simulink model "Australian14gen_original"  (R2017a)
settings: Solver=ode23tb  StartTime=0.0  StopTime=70  MaxStep=1/60  RelTol=1e-3  AbsTol=1e-1  EnableMultiTasking=on
PreLoadFcn:
  | dataaustralian14gen
values from neighbouring files (symbols this model uses):
  bus_v = [ 101	15 ... (first row only)    [dataaustralian14gen.m]
  comp = [ 1	211	0	0 ... (first row only)    [dataaustralian14gen.m]
  Exc = [ 101	0	 200	0.1	    13.25  2.5	 0	0       0       0       0       0 ... (first row only)    [dataaustralian14gen.m]
  FH = 13    [dataaustralian14gen.m]
  FI = 1    [dataaustralian14gen.m]
  FL = .1    (= 0.1)    [dataaustralian14gen.m]
  G_data = [ 101	333.3	15	3.6	0.14	1.1	0.65	0.25	8.5     0.25	0.05	0       0       0.25	0.2 	0 ... (first row only)    [dataaustralian14gen.m]
  KH = 120    [dataaustralian14gen.m]
  KI = 10    [dataaustralian14gen.m]
  KL = 10    [dataaustralian14gen.m]
  line = [ 102	217	0.0084	0.0667	0.817	330	1 ... (first row only)    [dataaustralian14gen.m]
  p = p_case4    [dataaustralian14gen.m]
  PSSMODEL = 1    [dataaustralian14gen.m]
  trans = [ 1	101	102	15	330	333.3	12	12 ... (first row only)    [dataaustralian14gen.m]
undefined symbols (not defined in the file or in its folder): D1, Delta
libraries: powerlib x297, sps_avr x14, factslib x5, powerlib_extras x4
(part 2 of 3)

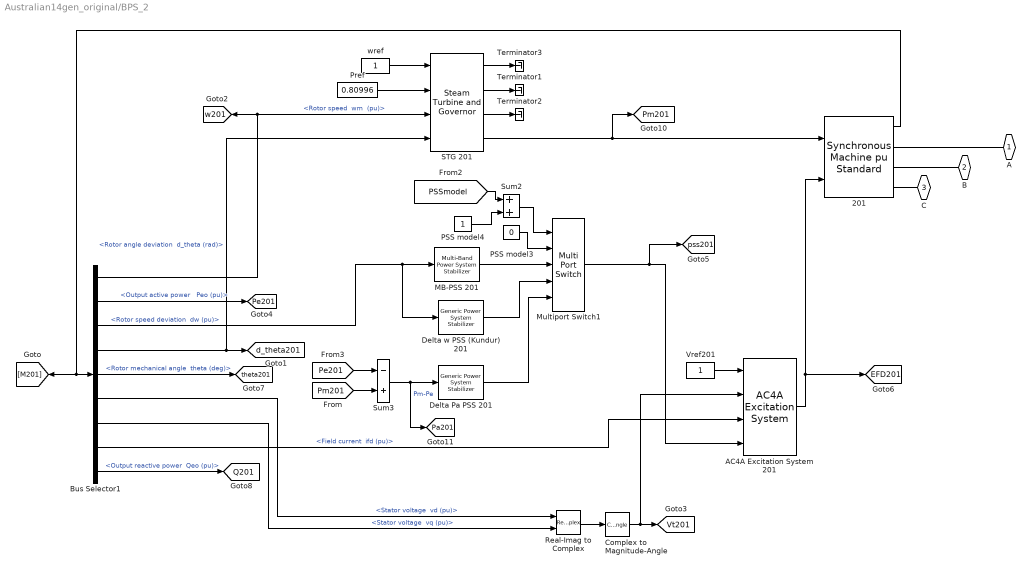
== system Australian14gen_original/BPS_2 ==
  201 : powerlib/Machines/Synchronous Machine pu Standard  PresetModel=No  MechanicalLoad=Mechanical power Pm  ShowDetailedParameters=on  RotorType=Round  Units=per unit standard parameters  MeasurementBus=off  NominalParameters="[G_data(2,2)*1e6  G_data(2,3)*1e3  50]"  Reactances1=[G_data(2,6),G_data(2,8),G_data(2,10),G_data(2,7),G_data(2,12),G_data(2,14),G_data(2,5)]  Reactances2=[G_data(2,6),G_data(2,8),G_data(2,10),G_data(2,7),G_data(2,14),G_data(2,5)]  dAxisTimeConstants=Open-circuit  qAxisTimeConstants=Open-circuit  TimeConstants1="[G_data(2,9)  G_data(2,11)  G_data(2,15)]"  TimeConstants2="[G_data(2,9), G_data(2,11), G_data(2,13),  G_data(2,15)]"  TimeConstants3="[  5.9  0.033  0.023  ]"  TimeConstants4=[ 8.0, 0.03, 0.3371, 0.0295 ]  TimeConstants5=[ 1.01, 0.053, 0.1 ]  TimeConstants6=[ 1.3201, 0.023, 1.0, 0.07 ]  TimeConstants7="[  1.01  0.053  0.051266  ]"  TimeConstants8=[ 1.3201, 0.0231, 0.3371, 0.0295 ]  StatorResistance=0  Mechanical="[ G_data(2,4) 0  4 ]"  PolePairs=4  InitialConditions=[0 -27.3285 0.811724 0.811724 0.811724 9.04729 -110.953 129.047 1.71513]  SetSaturation=off  Saturation=[0.6404,0.7127,0.8441,0.9214,0.9956,1.082,1.19,1.316,1.457;0.7,0.7698,0.8872,0.9466,0.9969,1.046,1.1,1.151,1.201]  LoadFlowParameters=[1 2160000000 20000 0 0]  TsPowergui=0  TsBlock=-1  IterativeModel=Forward Euler  IterativeDiscreteModel=Trapezoidal non iterative  BusType=PV  Pref=p(2,3)*1e6  Qref=0  Qmin=-inf  Qmax=inf  PLF=0  QLF=0
      settings: SourceProductName=Simscape Power Systems
  AC4A Excitation System 201 : sps_avr/AC4A Excitation System  Tr=Exc(2,2)  KaTa="[Exc(2,3)   Exc(2,4)]"  VIminmax=[-10 10]  VRminmax=[-4.53 5.64]  TbTc="[Exc(2,5)  Exc(2,6)]"  Kc=0  v0=[1 1.7151]  TsBlock=0
      settings: SourceProductName=Simscape Power Systems  SourceProductBaseCode=PS
  Bus Selector1 : BusSelector  OutputSignals="Mechanical.Rotor speed  wm  (pu),Output active power   Peo (pu),Mechanical.Rotor speed deviation  dw (pu),Mechanical.Rotor angle deviation  d_theta (rad),Mechanical.Rotor mechanical angle  theta (deg),dq0 components.Stator voltage  vd (pu),dq0 components.Stator voltage  vq (pu),dq0 components.Field current  ifd (pu),Output reactive power  Qeo (pu)"
  Complex to Magnitude-Angle : ComplexToMagnitudeAngle  Output=Magnitude
  Delta Pa PSS 201 : powerlib/Machines/Generic Power System Stabilizer  Tsensor=15e-3  K=2.5*1.25  Twashout=1  Tleadlag1=[60e-3 1]  Tleadlag2=[0 0]  VSlimits=[-0.15 0.15]  Vinit=0  Plot_On=off  MagdB_On=on  FreqRange=logspace(-2,2,500)
      settings: SourceProductName=Simscape Power Systems  SourceProductBaseCode=PS
  Delta w PSS (Kundur) 201 : powerlib/Machines/Generic Power System Stabilizer  Tsensor=15e-3  K=30  Twashout=10  Tleadlag1=[50e-3 20e-3]  Tleadlag2=[3 5.4]  VSlimits=[-0.15 0.15]  Vinit=0  Plot_On=off  MagdB_On=on  FreqRange=logspace(-2,2,500)
      settings: SourceProductName=Simscape Power Systems  SourceProductBaseCode=PS
  MB-PSS 201 : powerlib/Machines/Multi-Band Power System Stabilizer  OperationMode=Simplified settings  Kg=G  GL="[FL  KL]"  GI="[FI  KI]"  GH="[FH  KH]"  GLd=[66 66 9.4]  TcLF=[1.667 2 0 0 0 0 2 2.4 0 0 0 0 1 1]  GId=[66 66 47.6]  TcIF=[1 1 0.25 0.3 0 0 1 1 0.3 0.36 0 0 0 0]  GHd=[66 66 233]  TcHF="[0.01 0.012 0 0 0 0  0.012 0.0144 0 0 0 0 1 1]"  LIM=[.075 .15 .15 .15]  Plot_On=off  MagdB_On=off  FreqRange=logspace(-2,2,500)
      settings: SourceProductName=Simscape Power Systems  SourceProductBaseCode=PS
  Multiport Switch1 : MultiPortSwitch  Inputs=4  InputSameDT=on
  PSS model3 : Constant  Value=0
  PSS model4 : Constant
  Pref : Constant  Value=0.80996
  Real-Imag to Complex : RealImagToComplex
  STG 201 : powerlib/Machines/Steam Turbine and Governor  gentype=Tandem-compound (single mass)  reg1="[ 1  0.05    0 ]"  reg2="[ 0.001  0.15 ]"  reg3="[ -0.1  0.1  0  4.496 ]"  N=3000  turb1="[ 0  10   3.3   0.5   ]"  turb2="[   0   0.36    0.36   0.28   ]"  HA="[ 0.046  1.430  1.465   0.192 ]"  KA="[ 90.44  53.88  64.59   62.94  ]"  DA="[ 0.0115  0.3575  0.3663   0.0137  ]"  ini1=0.80996  ini2=[0.779316,-31.4247]
      settings: SourceProductName=Simscape Power Systems  SourceProductBaseCode=PS
  Sum2 : Sum  SaturateOnIntegerOverflow=on  InputSameDT=on  OutDataTypeStr=Inherit: Same as first input
  Sum3 : Sum  Inputs=-+  SaturateOnIntegerOverflow=on  InputSameDT=on  OutDataTypeStr=Inherit: Same as first input
  Terminator1 : Terminator
  Terminator2 : Terminator
  Terminator3 : Terminator
  Vref201 : Constant
  wref : Constant
  A : PMIOPort  Port=1  Side=Left
  B : PMIOPort  Port=2  Side=Left
  C : PMIOPort  Port=3  Side=Left
  tag scope: EFD201=global, Pa201=global, Pe201=global, Pm201=global, Q201=global, Vt201=global, d_theta201=global, pss201=global, theta201=global, w201=global
  wires:
  Bus Selector1/7 -> Real-Imag to Complex/2  "<Stator voltage  vq (pu)>"
  Bus Selector1/6 -> Real-Imag to Complex/1  "<Stator voltage  vd (pu)>"
  wref/1 -> STG 201/1
  Vref201/1 -> AC4A Excitation System 201/1
  Bus Selector1/4 -> STG 201/4, [d_theta201]  "<Rotor angle deviation  d_theta (rad)>"
  201/1 -> Bus Selector1/1, [M201]
  Bus Selector1/1 -> [w201], STG 201/3  "<Rotor speed  wm  (pu)>"
  Bus Selector1/3 -> Delta w PSS (Kundur) 201/1, MB-PSS 201/1  "<Rotor speed deviation  dw (pu)>"
  Real-Imag to Complex/1 -> Complex to Magnitude-Angle/1
  Complex to Magnitude-Angle/1 -> AC4A Excitation System 201/2, [Vt201]
  AC4A Excitation System 201/1 -> 201/2, [EFD201]
  Multiport Switch1/1 -> [pss201], AC4A Excitation System 201/4
  Bus Selector1/5 -> [theta201]  "<Rotor mechanical angle  theta (deg)>"
  Bus Selector1/2 -> [Pe201]  "<Output active power   Peo (pu)>"
  Bus Selector1/8 -> AC4A Excitation System 201/3  "<Field current  ifd (pu)>"
  Pref/1 -> STG 201/2
  STG 201/4 -> [Pm201], 201/1
  Bus Selector1/9 -> [Q201]  "<Output reactive power  Qeo (pu)>"
  PSS model4/1 -> Sum2/2
  Sum2/1 -> Multiport Switch1/1
  [PSSmodel] -> Sum2/1
  PSS model3/1 -> Multiport Switch1/2
  Sum3/1 -> [Pa201], Delta Pa PSS 201/1  "Pm-Pe"
  Delta Pa PSS 201/1 -> Multiport Switch1/5
  Delta w PSS (Kundur) 201/1 -> Multiport Switch1/4
  [Pm201] -> Sum3/2
  [Pe201] -> Sum3/1
  MB-PSS 201/1 -> Multiport Switch1/3
  STG 201/1 -> Terminator3/1
  STG 201/2 -> Terminator1/1
  STG 201/3 -> Terminator2/1
  connections:
  201/RConn1 -- A/RConn1
  201/RConn2 -- B/RConn1
  201/RConn3 -- C/RConn1

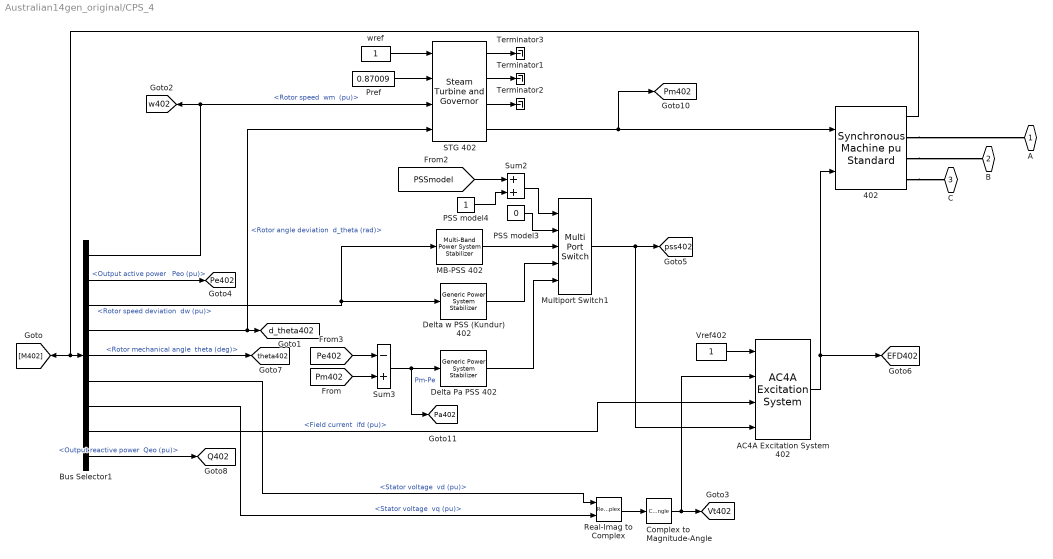
== system Australian14gen_original/CPS_4 ==
  402 : powerlib/Machines/Synchronous Machine pu Standard  PresetModel=No  MechanicalLoad=Mechanical power Pm  ShowDetailedParameters=on  RotorType=Round  Units=per unit standard parameters  MeasurementBus=off  NominalParameters="[G_data(9,2)*1e6  G_data(9,3)*1e3  50]"  Reactances1=[G_data(9,6),G_data(9,8),G_data(9,10),G_data(9,7),G_data(9,12),G_data(9,14),G_data(9,5)]  Reactances2=[G_data(9,6),G_data(9,8),G_data(9,10),G_data(9,7),G_data(9,14),G_data(9,5)]  dAxisTimeConstants=Open-circuit  qAxisTimeConstants=Open-circuit  TimeConstants1="[G_data(9,9)  G_data(9,11)  G_data(9,15)]"  TimeConstants2="[G_data(9,9)  G_data(9,11)  G_data(9,13)  G_data(9,15)]"  TimeConstants3="[  5.9  0.033  0.023  ]"  TimeConstants4=[ 8.0, 0.03, 0.3371, 0.0295 ]  TimeConstants5=[ 1.01, 0.053, 0.1 ]  TimeConstants6=[ 1.3201, 0.023, 1.0, 0.07 ]  TimeConstants7="[  1.01  0.053  0.051266  ]"  TimeConstants8=[ 1.3201, 0.0231, 0.3371, 0.0295 ]  StatorResistance=0  Mechanical="[ G_data(9,4) 0  4 ]"  PolePairs=4  InitialConditions=[0 -31.211 0.87022 0.87022 0.87022 1.63211 -118.368 121.632 1.91669]  SetSaturation=off  Saturation=[0.6404,0.7127,0.8441,0.9214,0.9956,1.082,1.19,1.316,1.457;0.7,0.7698,0.8872,0.9466,0.9969,1.046,1.1,1.151,1.201]  LoadFlowParameters=[1 580000000 20000 0 0]  TsPowergui=0  TsBlock=-1  IterativeModel=Forward Euler  IterativeDiscreteModel=Trapezoidal non iterative  BusType=PV  Pref=p(9,3)*1e6  Qref=0  Qmin=-inf  Qmax=inf  PLF=0  QLF=0
      settings: SourceProductName=Simscape Power Systems
  AC4A Excitation System 402 : sps_avr/AC4A Excitation System  Tr=Exc(9,2)  KaTa="[Exc(9,3)   Exc(9,4)]"  VIminmax=[-10 10]  VRminmax=[-4.53 5.64]  TbTc="[Exc(9,5)  Exc(9,6)]"  Kc=0  v0=[1 1.9167]  TsBlock=0
      settings: SourceProductName=Simscape Power Systems  SourceProductBaseCode=PS
  Bus Selector1 : BusSelector  OutputSignals="Mechanical.Rotor speed  wm  (pu),Output active power   Peo (pu),Mechanical.Rotor speed deviation  dw (pu),Mechanical.Rotor angle deviation  d_theta (rad),Mechanical.Rotor mechanical angle  theta (deg),dq0 components.Stator voltage  vd (pu),dq0 components.Stator voltage  vq (pu),dq0 components.Field current  ifd (pu),Output reactive power  Qeo (pu)"
  Complex to Magnitude-Angle : ComplexToMagnitudeAngle  Output=Magnitude
  Delta Pa PSS 402 : powerlib/Machines/Generic Power System Stabilizer  Tsensor=15e-3  K=2.5*1.25  Twashout=1  Tleadlag1=[60e-3 1]  Tleadlag2=[0 0]  VSlimits=[-0.15 0.15]  Vinit=0  Plot_On=off  MagdB_On=on  FreqRange=logspace(-2,2,500)
      settings: SourceProductName=Simscape Power Systems  SourceProductBaseCode=PS
  Delta w PSS (Kundur) 402 : powerlib/Machines/Generic Power System Stabilizer  Tsensor=15e-3  K=30  Twashout=10  Tleadlag1=[50e-3 20e-3]  Tleadlag2=[3 5.4]  VSlimits=[-0.15 0.15]  Vinit=0  Plot_On=off  MagdB_On=on  FreqRange=logspace(-2,2,500)
      settings: SourceProductName=Simscape Power Systems  SourceProductBaseCode=PS
  MB-PSS 402 : powerlib/Machines/Multi-Band Power System Stabilizer  OperationMode=Simplified settings  Kg=G  GL="[FL  KL]"  GI="[FI  KI]"  GH="[FH  KH]"  GLd=[66 66 9.4]  TcLF=[1.667 2 0 0 0 0 2 2.4 0 0 0 0 1 1]  GId=[66 66 47.6]  TcIF=[1 1 0.25 0.3 0 0 1 1 0.3 0.36 0 0 0 0]  GHd=[66 66 233]  TcHF="[0.01 0.012 0 0 0 0  0.012 0.0144 0 0 0 0 1 1]"  LIM=[.075 .15 .15 .15]  Plot_On=off  MagdB_On=off  FreqRange=logspace(-2,2,500)
      settings: SourceProductName=Simscape Power Systems  SourceProductBaseCode=PS
  Multiport Switch1 : MultiPortSwitch  Inputs=4  InputSameDT=on
  PSS model3 : Constant  Value=0
  PSS model4 : Constant
  Pref : Constant  Value=0.87009
  Real-Imag to Complex : RealImagToComplex
  STG 402 : powerlib/Machines/Steam Turbine and Governor  gentype=Tandem-compound (single mass)  reg1="[ 1  0.05    0 ]"  reg2="[ 0.001  0.15 ]"  reg3="[ -0.1  0.1  0  4.496 ]"  N=3000  turb1="[ 0  10   3.3   0.5   ]"  turb2="[   0   0.36    0.36   0.28   ]"  HA="[ 0.046  1.430  1.465   0.192 ]"  KA="[ 90.44  53.88  64.59   62.94  ]"  DA="[ 0.0115  0.3575  0.3663   0.0137  ]"  ini1=0.87009  ini2=[0.779316,-31.4247]
      settings: SourceProductName=Simscape Power Systems  SourceProductBaseCode=PS
  Sum2 : Sum  SaturateOnIntegerOverflow=on  InputSameDT=on  OutDataTypeStr=Inherit: Same as first input
  Sum3 : Sum  Inputs=-+  SaturateOnIntegerOverflow=on  InputSameDT=on  OutDataTypeStr=Inherit: Same as first input
  Terminator1 : Terminator
  Terminator2 : Terminator
  Terminator3 : Terminator
  Vref402 : Constant
  wref : Constant
  A : PMIOPort  Port=1  Side=Left
  B : PMIOPort  Port=2  Side=Left
  C : PMIOPort  Port=3  Side=Left
  tag scope: EFD402=global, Pa402=global, Pe402=global, Pm402=global, Q402=global, Vt402=global, d_theta402=global, pss402=global, theta402=global, w402=global
  wires:
  Bus Selector1/7 -> Real-Imag to Complex/2  "<Stator voltage  vq (pu)>"
  Bus Selector1/6 -> Real-Imag to Complex/1  "<Stator voltage  vd (pu)>"
  wref/1 -> STG 402/1
  Vref402/1 -> AC4A Excitation System 402/1
  Bus Selector1/4 -> STG 402/4, [d_theta402]  "<Rotor angle deviation  d_theta (rad)>"
  402/1 -> Bus Selector1/1, [M402]
  Bus Selector1/1 -> [w402], STG 402/3  "<Rotor speed  wm  (pu)>"
  Bus Selector1/3 -> Delta w PSS (Kundur) 402/1, MB-PSS 402/1  "<Rotor speed deviation  dw (pu)>"
  Real-Imag to Complex/1 -> Complex to Magnitude-Angle/1
  Complex to Magnitude-Angle/1 -> AC4A Excitation System 402/2, [Vt402]
  AC4A Excitation System 402/1 -> 402/2, [EFD402]
  Multiport Switch1/1 -> AC4A Excitation System 402/4, [pss402]
  Bus Selector1/5 -> [theta402]  "<Rotor mechanical angle  theta (deg)>"
  Bus Selector1/2 -> [Pe402]  "<Output active power   Peo (pu)>"
  Bus Selector1/8 -> AC4A Excitation System 402/3  "<Field current  ifd (pu)>"
  Pref/1 -> STG 402/2
  STG 402/4 -> [Pm402], 402/1
  Bus Selector1/9 -> [Q402]  "<Output reactive power  Qeo (pu)>"
  PSS model4/1 -> Sum2/2
  Sum2/1 -> Multiport Switch1/1
  [PSSmodel] -> Sum2/1
  PSS model3/1 -> Multiport Switch1/2
  Sum3/1 -> [Pa402], Delta Pa PSS 402/1  "Pm-Pe"
  Delta Pa PSS 402/1 -> Multiport Switch1/5
  Delta w PSS (Kundur) 402/1 -> Multiport Switch1/4
  [Pm402] -> Sum3/2
  [Pe402] -> Sum3/1
  MB-PSS 402/1 -> Multiport Switch1/3
  STG 402/1 -> Terminator3/1
  STG 402/2 -> Terminator1/1
  STG 402/3 -> Terminator2/1
  connections:
  402/RConn1 -- A/RConn1
  402/RConn2 -- B/RConn1
  402/RConn3 -- C/RConn1

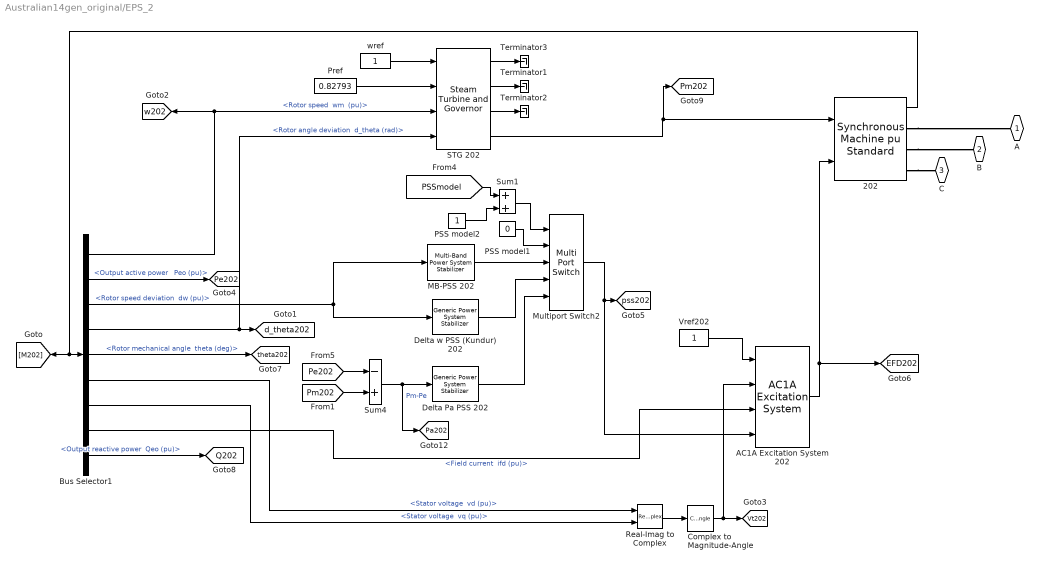
== system Australian14gen_original/EPS_2 ==
  202 : powerlib/Machines/Synchronous Machine pu Standard  PresetModel=No  MechanicalLoad=Mechanical power Pm  ShowDetailedParameters=on  RotorType=Round  Units=per unit standard parameters  MeasurementBus=off  NominalParameters="[G_data(3,2)*1e6  G_data(3,3)*1e3  50]"  Reactances1=[G_data(3,6),G_data(3,8),G_data(3,10),G_data(3,7),G_data(3,12), G_data(3,14),G_data(3,5)]  Reactances2=[G_data(3,6),G_data(3,8),G_data(3,10),G_data(3,7),G_data(3,12), G_data(3,14),G_data(3,5)]  dAxisTimeConstants=Open-circuit  qAxisTimeConstants=Open-circuit  TimeConstants1="[G_data(3,9)  G_data(3,11)  G_data(3,13) G_data(3,15)]"  TimeConstants2="[G_data(3,9)  G_data(3,11)  G_data(3,13) G_data(3,15)]"  TimeConstants3="[  5.9  0.033  0.023  ]"  TimeConstants4=[ 8.0, 0.03, 0.3371, 0.0295 ]  TimeConstants5=[ 1.01, 0.053, 0.1 ]  TimeConstants6=[ 1.3201, 0.023, 1.0, 0.07 ]  TimeConstants7="[  1.01  0.053  0.051266  ]"  TimeConstants8=[ 1.3201, 0.0231, 0.3371, 0.0295 ]  StatorResistance=0  Mechanical="[ G_data(3,4) 0  4 ]"  PolePairs=4  InitialConditions=[0 -27.8373 0.828196 0.828196 0.828196 2.41486 -117.585 122.415 2.0558]  SetSaturation=off  Saturation=[0.6404,0.7127,0.8441,0.9214,0.9956,1.082,1.19,1.316,1.457;0.7,0.7698,0.8872,0.9466,0.9969,1.046,1.1,1.151,1.201]  LoadFlowParameters=[1 1380000000 20000 0 0]  TsPowergui=0  TsBlock=-1  IterativeModel=Forward Euler  IterativeDiscreteModel=Trapezoidal non iterative  BusType=PV  Pref=p(3,3)*1e6  Qref=0  Qmin=-inf  Qmax=inf  PLF=0  QLF=0
      settings: SourceProductName=Simscape Power Systems
  AC1A Excitation System 202 : sps_avr/AC1A Excitation System  Tr=Exc(3,2)  KaTa="[Exc(3,3)   Exc(3,4)]"  VAminmax=[-14.5 14.5]  VRminmax=[-5.43 6.03]  KfTf="[Exc(3,9)  Exc(3,10)]"  TbTc="[Exc(3,5)  Exc(3,6)]"  KeTe="[Exc(3,7)  Exc(3,8)]"  Ve12=[4.18 3.14]  SeVe12=[0.10 0.03]  Kd=0.38  Kc=0.20  v0=[1 2.0558]  TsBlock=0
      settings: SourceProductName=Simscape Power Systems  SourceProductBaseCode=PS
  Bus Selector1 : BusSelector  OutputSignals="Mechanical.Rotor speed  wm  (pu),Output active power   Peo (pu),Mechanical.Rotor speed deviation  dw (pu),Mechanical.Rotor angle deviation  d_theta (rad),Mechanical.Rotor mechanical angle  theta (deg),dq0 components.Stator voltage  vd (pu),dq0 components.Stator voltage  vq (pu),dq0 components.Field current  ifd (pu),Output reactive power  Qeo (pu)"
  Complex to Magnitude-Angle : ComplexToMagnitudeAngle  Output=Magnitude
  Delta Pa PSS 202 : powerlib/Machines/Generic Power System Stabilizer  Tsensor=15e-3  K=2.5*1.25  Twashout=1  Tleadlag1=[60e-3 1]  Tleadlag2=[0 0]  VSlimits=[-0.15 0.15]  Vinit=0  Plot_On=off  MagdB_On=on  FreqRange=logspace(-2,2,500)
      settings: SourceProductName=Simscape Power Systems  SourceProductBaseCode=PS
  Delta w PSS (Kundur) 202 : powerlib/Machines/Generic Power System Stabilizer  Tsensor=15e-3  K=30  Twashout=10  Tleadlag1=[50e-3 20e-3]  Tleadlag2=[3 5.4]  VSlimits=[-0.15 0.15]  Vinit=0  Plot_On=off  MagdB_On=on  FreqRange=logspace(-2,2,500)
      settings: SourceProductName=Simscape Power Systems  SourceProductBaseCode=PS
  MB-PSS 202 : powerlib/Machines/Multi-Band Power System Stabilizer  OperationMode=Simplified settings  Kg=G  GL="[FL  KL]"  GI="[FI  KI]"  GH="[FH  KH]"  GLd=[66 66 9.4]  TcLF=[1.667 2 0 0 0 0 2 2.4 0 0 0 0 1 1]  GId=[66 66 47.6]  TcIF=[1 1 0.25 0.3 0 0 1 1 0.3 0.36 0 0 0 0]  GHd=[66 66 233]  TcHF="[0.01 0.012 0 0 0 0  0.012 0.0144 0 0 0 0 1 1]"  LIM=[.075 .15 .15 .15]  Plot_On=off  MagdB_On=off  FreqRange=logspace(-2,2,500)
      settings: SourceProductName=Simscape Power Systems  SourceProductBaseCode=PS
  Multiport Switch2 : MultiPortSwitch  Inputs=4  InputSameDT=on
  PSS model1 : Constant  Value=0
  PSS model2 : Constant
  Pref : Constant  Value=0.82793
  Real-Imag to Complex : RealImagToComplex
  STG 202 : powerlib/Machines/Steam Turbine and Governor  gentype=Tandem-compound (single mass)  reg1="[ 1  0.05    0 ]"  reg2="[ 0.001  0.15 ]"  reg3="[ -0.1  0.1  0  4.496 ]"  N=3000  turb1="[ 0  10   3.3   0.5   ]"  turb2="[   0   0.36    0.36   0.28   ]"  HA="[ 0.046  1.430  1.465   0.192 ]"  KA="[ 90.44  53.88  64.59   62.94  ]"  DA="[ 0.0115  0.3575  0.3663   0.0137  ]"  ini1=0.82793  ini2=[0.779316,-31.4247]
      settings: SourceProductName=Simscape Power Systems  SourceProductBaseCode=PS
  Sum1 : Sum  SaturateOnIntegerOverflow=on  InputSameDT=on  OutDataTypeStr=Inherit: Same as first input
  Sum4 : Sum  Inputs=-+  SaturateOnIntegerOverflow=on  InputSameDT=on  OutDataTypeStr=Inherit: Same as first input
  Terminator1 : Terminator
  Terminator2 : Terminator
  Terminator3 : Terminator
  Vref202 : Constant
  wref : Constant
  A : PMIOPort  Port=1  Side=Left
  B : PMIOPort  Port=2  Side=Left
  C : PMIOPort  Port=3  Side=Left
  tag scope: EFD202=global, Pa202=global, Pe202=global, Pm202=global, Q202=global, Vt202=global, d_theta202=global, pss202=global, theta202=global, w202=global
  wires:
  Bus Selector1/7 -> Real-Imag to Complex/2  "<Stator voltage  vq (pu)>"
  Bus Selector1/6 -> Real-Imag to Complex/1  "<Stator voltage  vd (pu)>"
  wref/1 -> STG 202/1
  Vref202/1 -> AC1A Excitation System 202/1
  Bus Selector1/4 -> STG 202/4, [d_theta202]  "<Rotor angle deviation  d_theta (rad)>"
  202/1 -> [M202], Bus Selector1/1
  Bus Selector1/1 -> STG 202/3, [w202]  "<Rotor speed  wm  (pu)>"
  Bus Selector1/3 -> MB-PSS 202/1, Delta w PSS (Kundur) 202/1  "<Rotor speed deviation  dw (pu)>"
  Real-Imag to Complex/1 -> Complex to Magnitude-Angle/1
  Complex to Magnitude-Angle/1 -> AC1A Excitation System 202/2, [Vt202]
  AC1A Excitation System 202/1 -> 202/2, [EFD202]
  Multiport Switch2/1 -> AC1A Excitation System 202/4, [pss202]
  Bus Selector1/5 -> [theta202]  "<Rotor mechanical angle  theta (deg)>"
  Bus Selector1/2 -> [Pe202]  "<Output active power   Peo (pu)>"
  Bus Selector1/8 -> AC1A Excitation System 202/3  "<Field current  ifd (pu)>"
  Pref/1 -> STG 202/2
  STG 202/4 -> [Pm202], 202/1
  Bus Selector1/9 -> [Q202]  "<Output reactive power  Qeo (pu)>"
  PSS model2/1 -> Sum1/2
  Sum1/1 -> Multiport Switch2/1
  [PSSmodel] -> Sum1/1
  PSS model1/1 -> Multiport Switch2/2
  Sum4/1 -> [Pa202], Delta Pa PSS 202/1  "Pm-Pe"
  Delta Pa PSS 202/1 -> Multiport Switch2/5
  Delta w PSS (Kundur) 202/1 -> Multiport Switch2/4
  [Pm202] -> Sum4/2
  [Pe202] -> Sum4/1
  MB-PSS 202/1 -> Multiport Switch2/3
  STG 202/1 -> Terminator3/1
  STG 202/2 -> Terminator1/1
  STG 202/3 -> Terminator2/1
  connections:
  202/RConn1 -- A/RConn1
  202/RConn2 -- B/RConn1
  202/RConn3 -- C/RConn1

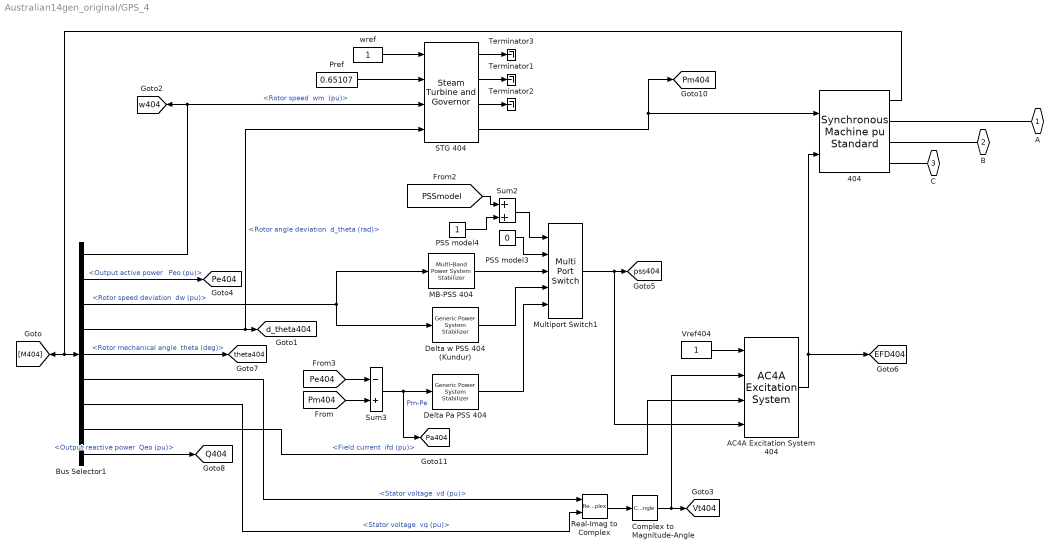
== system Australian14gen_original/GPS_4 ==
  404 : powerlib/Machines/Synchronous Machine pu Standard  PresetModel=No  MechanicalLoad=Mechanical power Pm  ShowDetailedParameters=on  RotorType=Round  Units=per unit standard parameters  MeasurementBus=off  NominalParameters="[G_data(11,2)*1e6  G_data(11,3)*1e3  50]"  Reactances1="[G_data(11,6),G_data(11,8),G_data(11,10),G_data(11,7),  G_data(11,12),G_data(11,14),G_data(11,5)]"  Reactances2="[G_data(11,6),G_data(11,8),G_data(11,10),G_data(11,7),  G_data(11,12),G_data(11,14),G_data(11,5)]"  dAxisTimeConstants=Open-circuit  qAxisTimeConstants=Open-circuit  TimeConstants1="[G_data(11,9)  G_data(11,11)   G_data(11,13) G_data(11,15)]"  TimeConstants2="[G_data(11,9)  G_data(11,11)   G_data(11,13)  G_data(11,15)]"  TimeConstants3="[  5.9  0.033  0.023  ]"  TimeConstants4=[ 8.0, 0.03, 0.3371, 0.0295 ]  TimeConstants5=[ 1.01, 0.053, 0.1 ]  TimeConstants6=[ 1.3201, 0.023, 1.0, 0.07 ]  TimeConstants7="[  1.01  0.053  0.051266  ]"  TimeConstants8=[ 1.3201, 0.0231, 0.3371, 0.0295 ]  StatorResistance=0  Mechanical="[ G_data(11,4) 0  4 ]"  PolePairs=4  InitialConditions=[0 -53.1224 0.651374 0.651374 0.651374 -4.51974 -124.52 115.48 1.67704]  SetSaturation=off  Saturation=[0.6404,0.7127,0.8441,0.9214,0.9956,1.082,1.19,1.316,1.457;0.7,0.7698,0.8872,0.9466,0.9969,1.046,1.1,1.151,1.201]  LoadFlowParameters=[1 651000000 20000 0 0]  TsPowergui=0  TsBlock=-1  IterativeModel=Forward Euler  IterativeDiscreteModel=Trapezoidal non iterative  BusType=PV  Pref=p(11,3)*1e6  Qref=0  Qmin=-inf  Qmax=inf  PLF=0  QLF=0
      settings: SourceProductName=Simscape Power Systems
  AC4A Excitation System 404 : sps_avr/AC4A Excitation System  Tr=Exc(11,2)  KaTa="[Exc(11,3)   Exc(11,4)]"  VIminmax=[-10 10]  VRminmax=[-4.53 5.64]  TbTc="[Exc(11,5)  Exc(11,6)]"  Kc=0  v0=[1 1.677]  TsBlock=0
      settings: SourceProductName=Simscape Power Systems  SourceProductBaseCode=PS
  Bus Selector1 : BusSelector  OutputSignals="Mechanical.Rotor speed  wm  (pu),Output active power   Peo (pu),Mechanical.Rotor speed deviation  dw (pu),Mechanical.Rotor angle deviation  d_theta (rad),Mechanical.Rotor mechanical angle  theta (deg),dq0 components.Stator voltage  vd (pu),dq0 components.Stator voltage  vq (pu),dq0 components.Field current  ifd (pu),Output reactive power  Qeo (pu)"
  Complex to Magnitude-Angle : ComplexToMagnitudeAngle  Output=Magnitude
  "Delta Pa PSS 404 " : powerlib/Machines/Generic Power System Stabilizer  Tsensor=15e-3  K=2.5*1.25  Twashout=1  Tleadlag1=[60e-3 1]  Tleadlag2=[0 0]  VSlimits=[-0.15 0.15]  Vinit=0  Plot_On=off  MagdB_On=on  FreqRange=logspace(-2,2,500)
      settings: SourceProductName=Simscape Power Systems  SourceProductBaseCode=PS
  "Delta w PSS 404 (Kundur) " : powerlib/Machines/Generic Power System Stabilizer  Tsensor=15e-3  K=30  Twashout=10  Tleadlag1=[50e-3 20e-3]  Tleadlag2=[3 5.4]  VSlimits=[-0.15 0.15]  Vinit=0  Plot_On=off  MagdB_On=on  FreqRange=logspace(-2,2,500)
      settings: SourceProductName=Simscape Power Systems  SourceProductBaseCode=PS
  "MB-PSS 404 " : powerlib/Machines/Multi-Band Power System Stabilizer  OperationMode=Simplified settings  Kg=G  GL="[FL  KL]"  GI="[FI  KI]"  GH="[FH  KH]"  GLd=[66 66 9.4]  TcLF=[1.667 2 0 0 0 0 2 2.4 0 0 0 0 1 1]  GId=[66 66 47.6]  TcIF=[1 1 0.25 0.3 0 0 1 1 0.3 0.36 0 0 0 0]  GHd=[66 66 233]  TcHF="[0.01 0.012 0 0 0 0  0.012 0.0144 0 0 0 0 1 1]"  LIM=[.075 .15 .15 .15]  Plot_On=off  MagdB_On=off  FreqRange=logspace(-2,2,500)
      settings: SourceProductName=Simscape Power Systems  SourceProductBaseCode=PS
  Multiport Switch1 : MultiPortSwitch  Inputs=4  InputSameDT=on
  PSS model3 : Constant  Value=0
  PSS model4 : Constant
  Pref : Constant  Value=0.65107
  Real-Imag to Complex : RealImagToComplex
  STG 404 : powerlib/Machines/Steam Turbine and Governor  gentype=Tandem-compound (single mass)  reg1="[ 1  0.05    0 ]"  reg2="[ 0.001  0.15 ]"  reg3="[ -0.1  0.1  0  4.496 ]"  N=3000  turb1="[ 0  10   3.3   0.5   ]"  turb2="[   0   0.36    0.36   0.28   ]"  HA="[ 0.046  1.430  1.465   0.192 ]"  KA="[ 90.44  53.88  64.59   62.94  ]"  DA="[ 0.0115  0.3575  0.3663   0.0137  ]"  ini1=0.65107  ini2=[0.779316,-31.4247]
      settings: SourceProductName=Simscape Power Systems  SourceProductBaseCode=PS
  Sum2 : Sum  SaturateOnIntegerOverflow=on  InputSameDT=on  OutDataTypeStr=Inherit: Same as first input
  Sum3 : Sum  Inputs=-+  SaturateOnIntegerOverflow=on  InputSameDT=on  OutDataTypeStr=Inherit: Same as first input
  Terminator1 : Terminator
  Terminator2 : Terminator
  Terminator3 : Terminator
  Vref404 : Constant
  wref : Constant
  A : PMIOPort  Port=1  Side=Left
  B : PMIOPort  Port=2  Side=Left
  C : PMIOPort  Port=3  Side=Left
  tag scope: EFD404=global, Pa404=global, Pe404=global, Pm404=global, Q404=global, Vt404=global, d_theta404=global, pss404=global, theta404=global, w404=global
  wires:
  Bus Selector1/7 -> Real-Imag to Complex/2  "<Stator voltage  vq (pu)>"
  Bus Selector1/6 -> Real-Imag to Complex/1  "<Stator voltage  vd (pu)>"
  wref/1 -> STG 404/1
  Vref404/1 -> AC4A Excitation System 404/1
  Bus Selector1/4 -> STG 404/4, [d_theta404]  "<Rotor angle deviation  d_theta (rad)>"
  404/1 -> [M404], Bus Selector1/1
  Bus Selector1/1 -> [w404], STG 404/3  "<Rotor speed  wm  (pu)>"
  Bus Selector1/3 -> "MB-PSS 404 "/1, "Delta w PSS 404 (Kundur) "/1  "<Rotor speed deviation  dw (pu)>"
  Real-Imag to Complex/1 -> Complex to Magnitude-Angle/1
  Complex to Magnitude-Angle/1 -> AC4A Excitation System 404/2, [Vt404]
  AC4A Excitation System 404/1 -> 404/2, [EFD404]
  Multiport Switch1/1 -> AC4A Excitation System 404/4, [pss404]
  Bus Selector1/5 -> [theta404]  "<Rotor mechanical angle  theta (deg)>"
  Bus Selector1/2 -> [Pe404]  "<Output active power   Peo (pu)>"
  Bus Selector1/8 -> AC4A Excitation System 404/3  "<Field current  ifd (pu)>"
  Pref/1 -> STG 404/2
  STG 404/4 -> [Pm404], 404/1
  Bus Selector1/9 -> [Q404]  "<Output reactive power  Qeo (pu)>"
  PSS model4/1 -> Sum2/2
  Sum2/1 -> Multiport Switch1/1
  [PSSmodel] -> Sum2/1
  PSS model3/1 -> Multiport Switch1/2
  Sum3/1 -> [Pa404], "Delta Pa PSS 404 "/1  "Pm-Pe"
  "Delta Pa PSS 404 "/1 -> Multiport Switch1/5
  "Delta w PSS 404 (Kundur) "/1 -> Multiport Switch1/4
  [Pm404] -> Sum3/2
  [Pe404] -> Sum3/1
  "MB-PSS 404 "/1 -> Multiport Switch1/3
  STG 404/1 -> Terminator3/1
  STG 404/2 -> Terminator1/1
  STG 404/3 -> Terminator2/1
  connections:
  404/RConn1 -- A/RConn1
  404/RConn2 -- B/RConn1
  404/RConn3 -- C/RConn1

== system Australian14gen_original/HPS_1 ==
  101 : powerlib/Machines/Synchronous Machine pu Standard  PresetModel=No  MechanicalLoad=Mechanical power Pm  ShowDetailedParameters=on  RotorType=Round  Units=per unit standard parameters  MeasurementBus=off  NominalParameters="[G_data(1,2)*1e6  G_data(1,3)*1e3  50]"  Reactances1="[G_data(1,6),G_data(1,8),G_data(1,10),G_data(1,7),  G_data(1,12),G_data(1,14),G_data(1,5)]"  Reactances2=[G_data(1,6),G_data(1,8),G_data(1,10),G_data(1,7),G_data(1,12),G_data(1,14),G_data(1,5)]  dAxisTimeConstants=Open-circuit  qAxisTimeConstants=Open-circuit  TimeConstants1="[G_data(1,9)  G_data(1,11)  G_data(1,13)  G_data(1,15)]"  TimeConstants2="[G_data(1,9)  G_data(1,11)   G_data(1,13)  G_data(1,15)]"  TimeConstants3="[  5.9  0.033  0.023  ]"  TimeConstants4="[G_data(1,9)  G_data(1,11)   G_data(1,13)  G_data(1,15)]"  TimeConstants5=[ 1.01, 0.053, 0.1 ]  TimeConstants6=[ 1.3201, 0.023, 1.0, 0.07 ]  TimeConstants7="[  1.01  0.053  0.051266  ]"  TimeConstants8=[ 1.3201, 0.0231, 0.3371, 0.0295 ]  StatorResistance=0  Mechanical="[ G_data(1,4) 0  4 ]"  PolePairs=4  InitialConditions=[0 -112.344 0.314975 0.314975 0.314975 67.656 -52.344 187.656 0.653527]  SetSaturation=off  Saturation=[0.6404,0.7127,0.8441,0.9214,0.9956,1.082,1.19,1.316,1.457;0.7,0.7698,0.8872,0.9466,0.9969,1.046,1.1,1.151,1.201]  LoadFlowParameters=[1 1000 15000 0 0]  TsPowergui=0  TsBlock=-1  IterativeModel=Forward Euler  IterativeDiscreteModel=Trapezoidal non iterative  BusType=PV  Pref=1000  Qref=0  Qmin=-inf  Qmax=inf  PLF=0  QLF=0
      settings: SourceProductName=Simscape Power Systems
  AC4A Excitation System 101 : sps_avr/AC4A Excitation System  Tr=Exc(1,2)  KaTa="[Exc(1,3)   Exc(1,4)]"  VIminmax=[-10 10]  VRminmax=[-4.53 5.64]  TbTc="[Exc(1,5)  Exc(1,6)]"  Kc=0  v0=[1 0.65353]  TsBlock=0
      settings: SourceProductName=Simscape Power Systems  SourceProductBaseCode=PS
  Bus Selector1 : BusSelector  OutputSignals="Mechanical.Rotor speed  wm  (pu),Output active power   Peo (pu),Mechanical.Rotor speed deviation  dw (pu),Mechanical.Rotor angle deviation  d_theta (rad),Mechanical.Rotor mechanical angle  theta (deg),dq0 components.Stator voltage  vd (pu),dq0 components.Stator voltage  vq (pu),dq0 components.Field current  ifd (pu),Output reactive power  Qeo (pu)"
  Complex to Magnitude-Angle : ComplexToMagnitudeAngle  Output=Magnitude
  Delta Pa PSS  101 : powerlib/Machines/Generic Power System Stabilizer  Tsensor=15e-3  K=2.5*1.25  Twashout=1  Tleadlag1=[60e-3 1]  Tleadlag2=[0 0]  VSlimits=[-0.15 0.15]  Vinit=0  Plot_On=off  MagdB_On=on  FreqRange=logspace(-2,2,500)
      settings: SourceProductName=Simscape Power Systems  SourceProductBaseCode=PS
  Delta w PSS (Kundur)  101 : powerlib/Machines/Generic Power System Stabilizer  Tsensor=15e-3  K=30  Twashout=10  Tleadlag1=[50e-3 20e-3]  Tleadlag2=[3 5.4]  VSlimits=[-0.15 0.15]  Vinit=0  Plot_On=off  MagdB_On=on  FreqRange=logspace(-2,2,500)
      settings: SourceProductName=Simscape Power Systems  SourceProductBaseCode=PS
  MB-PSS  101 : powerlib/Machines/Multi-Band Power System Stabilizer  OperationMode=Simplified settings  Kg=G  GL="[FL  KL]"  GI="[FI  KI]"  GH="[FH  KH]"  GLd=[66 66 9.4]  TcLF=[1.667 2 0 0 0 0 2 2.4 0 0 0 0 1 1]  GId=[66 66 47.6]  TcIF=[1 1 0.25 0.3 0 0 1 1 0.3 0.36 0 0 0 0]  GHd=[66 66 233]  TcHF="[0.01 0.012 0 0 0 0  0.012 0.0144 0 0 0 0 1 1]"  LIM=[.075 .15 .15 .15]  Plot_On=off  MagdB_On=off  FreqRange=logspace(-2,2,500)
      settings: SourceProductName=Simscape Power Systems  SourceProductBaseCode=PS
  Multiport Switch1 : MultiPortSwitch  Inputs=4  InputSameDT=on
  PSS model3 : Constant  Value=0
  PSS model4 : Constant
  Pref : Constant  Value=1.5002e-06
  Real-Imag to Complex : RealImagToComplex
  Sum2 : Sum  SaturateOnIntegerOverflow=on  InputSameDT=on  OutDataTypeStr=Inherit: Same as first input
  Sum3 : Sum  Inputs=-+  SaturateOnIntegerOverflow=on  InputSameDT=on  OutDataTypeStr=Inherit: Same as first input
  Vref101 : Constant
  A : PMIOPort  Port=1  Side=Left
  B : PMIOPort  Port=2  Side=Left
  C : PMIOPort  Port=3  Side=Left
  tag scope: EFD101=global, Pa101=global, Pe101=global, Pm101=global, Q101=global, Vt101=global, d_theta101=global, pss101=global, theta101=global, w101=global
  wires:
  Bus Selector1/7 -> Real-Imag to Complex/2  "<Stator voltage  vq (pu)>"
  Bus Selector1/6 -> Real-Imag to Complex/1  "<Stator voltage  vd (pu)>"
  Vref101/1 -> AC4A Excitation System 101/1
  Bus Selector1/4 -> [d_theta101]  "<Rotor angle deviation  d_theta (rad)>"
  101/1 -> Bus Selector1/1, [M101]
  Bus Selector1/1 -> [w101]  "<Rotor speed  wm  (pu)>"
  Bus Selector1/3 -> Delta w PSS (Kundur)  101/1, MB-PSS  101/1  "<Rotor speed deviation  dw (pu)>"
  Real-Imag to Complex/1 -> Complex to Magnitude-Angle/1
  AC4A Excitation System 101/1 -> 101/2, [EFD101]
  Multiport Switch1/1 -> [pss101], AC4A Excitation System 101/4
  Bus Selector1/5 -> [theta101]  "<Rotor mechanical angle  theta (deg)>"
  Bus Selector1/2 -> [Pe101]  "<Output active power   Peo (pu)>"
  Bus Selector1/8 -> AC4A Excitation System 101/3  "<Field current  ifd (pu)>"
  Complex to Magnitude-Angle/1 -> AC4A Excitation System 101/2, [Vt101]
  Pref/1 -> [Pm101], 101/1
  Bus Selector1/9 -> [Q101]  "<Output reactive power  Qeo (pu)>"
  PSS model4/1 -> Sum2/2
  Sum2/1 -> Multiport Switch1/1
  [PSSmodel] -> Sum2/1
  PSS model3/1 -> Multiport Switch1/2
  Sum3/1 -> [Pa101], Delta Pa PSS  101/1  "Pm-Pe"
  Delta Pa PSS  101/1 -> Multiport Switch1/5
  Delta w PSS (Kundur)  101/1 -> Multiport Switch1/4
  [Pm101] -> Sum3/2
  [Pe101] -> Sum3/1
  MB-PSS  101/1 -> Multiport Switch1/3
  connections:
  101/RConn1 -- A/RConn1
  101/RConn2 -- B/RConn1
  101/RConn3 -- C/RConn1

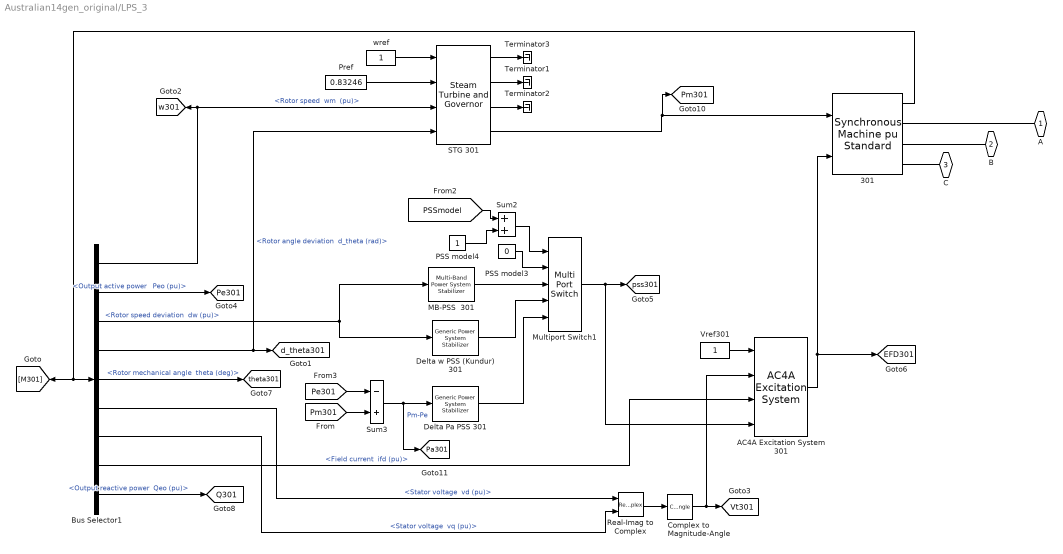
== system Australian14gen_original/LPS_3 ==
  301 : powerlib/Machines/Synchronous Machine pu Standard  PresetModel=No  MechanicalLoad=Mechanical power Pm  ShowDetailedParameters=on  RotorType=Round  Units=per unit standard parameters  MeasurementBus=off  NominalParameters="[G_data(6,2)*1E6  G_data(6,3)*1E3  50]"  Reactances1=[G_data(6,6),G_data(6,8),G_data(6,10),G_data(6,7),G_data(6,12),G_data(6,14),G_data(6,5)]  Reactances2=[G_data(6,6),G_data(6,8),G_data(6,10),G_data(6,7),G_data(6,12),G_data(6,14),G_data(6,5)]  dAxisTimeConstants=Open-circuit  qAxisTimeConstants=Open-circuit  TimeConstants1="[G_data(6,9)  G_data(6,11)  G_data(6,13)  G_data(6,15)]"  TimeConstants2="[G_data(6,9)  G_data(6,11)  G_data(6,13)  G_data(6,15)]"  TimeConstants3="[  5.9  0.033  0.023  ]"  TimeConstants4=[ 8.0, 0.03, 0.3371, 0.0295 ]  TimeConstants5=[ 1.01, 0.053, 0.1 ]  TimeConstants6=[ 1.3201, 0.023, 1.0, 0.07 ]  TimeConstants7="[  1.01  0.053  0.051266  ]"  TimeConstants8=[ 1.3201, 0.0231, 0.3371, 0.0295 ]  StatorResistance=0  Mechanical="[ G_data(6,4) 0  4 ]"  PolePairs=4  InitialConditions=[0 -48.0444 0.832693 0.832693 0.832693 -9.89662 -129.897 110.103 2.40429]  SetSaturation=off  Saturation=[0.6404,0.7127,0.8441,0.9214,0.9956,1.082,1.19,1.316,1.457;0.7,0.7698,0.8872,0.9466,0.9969,1.046,1.1,1.151,1.201]  LoadFlowParameters=[1 3330000000 20000 0 0]  TsPowergui=0  TsBlock=-1  IterativeModel=Forward Euler  IterativeDiscreteModel=Trapezoidal non iterative  BusType=PV  Pref=p(6,3)*1e6  Qref=0  Qmin=-inf  Qmax=inf  PLF=0  QLF=0
      settings: SourceProductName=Simscape Power Systems
  AC4A Excitation System 301 : sps_avr/AC4A Excitation System  Tr=Exc(6,2)  KaTa="[Exc(6,3)   Exc(6,4)]"  VIminmax=[-10 10]  VRminmax=[-4.53 5.64]  TbTc="[Exc(6,5)  Exc(6,6)]"  Kc=0  v0=[1 2.4043]  TsBlock=0
      settings: SourceProductName=Simscape Power Systems  SourceProductBaseCode=PS
  Bus Selector1 : BusSelector  OutputSignals="Mechanical.Rotor speed  wm  (pu),Output active power   Peo (pu),Mechanical.Rotor speed deviation  dw (pu),Mechanical.Rotor angle deviation  d_theta (rad),Mechanical.Rotor mechanical angle  theta (deg),dq0 components.Stator voltage  vd (pu),dq0 components.Stator voltage  vq (pu),dq0 components.Field current  ifd (pu),Output reactive power  Qeo (pu)"
  Complex to Magnitude-Angle : ComplexToMagnitudeAngle  Output=Magnitude
  "Delta Pa PSS 301 " : powerlib/Machines/Generic Power System Stabilizer  Tsensor=15e-3  K=2.5*1.25  Twashout=1  Tleadlag1=[60e-3 1]  Tleadlag2=[0 0]  VSlimits=[-0.15 0.15]  Vinit=0  Plot_On=off  MagdB_On=on  FreqRange=logspace(-2,2,500)
      settings: SourceProductName=Simscape Power Systems  SourceProductBaseCode=PS
  "Delta w PSS (Kundur) 301 " : powerlib/Machines/Generic Power System Stabilizer  Tsensor=15e-3  K=30  Twashout=10  Tleadlag1=[50e-3 20e-3]  Tleadlag2=[3 5.4]  VSlimits=[-0.15 0.15]  Vinit=0  Plot_On=off  MagdB_On=on  FreqRange=logspace(-2,2,500)
      settings: SourceProductName=Simscape Power Systems  SourceProductBaseCode=PS
  MB-PSS  301 : powerlib/Machines/Multi-Band Power System Stabilizer  OperationMode=Simplified settings  Kg=G  GL="[FL  KL]"  GI="[FI  KI]"  GH="[FH  KH]"  GLd=[66 66 9.4]  TcLF=[1.667 2 0 0 0 0 2 2.4 0 0 0 0 1 1]  GId=[66 66 47.6]  TcIF=[1 1 0.25 0.3 0 0 1 1 0.3 0.36 0 0 0 0]  GHd=[66 66 233]  TcHF="[0.01 0.012 0 0 0 0  0.012 0.0144 0 0 0 0 1 1]"  LIM=[.075 .15 .15 .15]  Plot_On=off  MagdB_On=off  FreqRange=logspace(-2,2,500)
      settings: SourceProductName=Simscape Power Systems  SourceProductBaseCode=PS
  Multiport Switch1 : MultiPortSwitch  Inputs=4  InputSameDT=on
  PSS model3 : Constant  Value=0
  PSS model4 : Constant
  Pref : Constant  Value=0.83246
  Real-Imag to Complex : RealImagToComplex
  STG 301 : powerlib/Machines/Steam Turbine and Governor  gentype=Tandem-compound (single mass)  reg1="[ 1  0.05    0 ]"  reg2="[ 0.001  0.15 ]"  reg3="[ -0.1  0.1  0  4.496 ]"  N=3000  turb1="[ 0  10   3.3   0.5   ]"  turb2="[   0   0.36    0.36   0.28   ]"  HA="[ 0.046  1.430  1.465   0.192 ]"  KA="[ 90.44  53.88  64.59   62.94  ]"  DA="[ 0.0115  0.3575  0.3663   0.0137  ]"  ini1=0.83246  ini2=[0.779316,-31.4247]
      settings: SourceProductName=Simscape Power Systems  SourceProductBaseCode=PS
  Sum2 : Sum  SaturateOnIntegerOverflow=on  InputSameDT=on  OutDataTypeStr=Inherit: Same as first input
  Sum3 : Sum  Inputs=-+  SaturateOnIntegerOverflow=on  InputSameDT=on  OutDataTypeStr=Inherit: Same as first input
  Terminator1 : Terminator
  Terminator2 : Terminator
  Terminator3 : Terminator
  Vref301 : Constant
  wref : Constant
  A : PMIOPort  Port=1  Side=Left
  B : PMIOPort  Port=2  Side=Left
  C : PMIOPort  Port=3  Side=Left
  tag scope: EFD301=global, Pa301=global, Pe301=global, Pm301=global, Q301=global, Vt301=global, d_theta301=global, pss301=global, theta301=global, w301=global
  wires:
  Bus Selector1/7 -> Real-Imag to Complex/2  "<Stator voltage  vq (pu)>"
  Bus Selector1/6 -> Real-Imag to Complex/1  "<Stator voltage  vd (pu)>"
  wref/1 -> STG 301/1
  Vref301/1 -> AC4A Excitation System 301/1
  Bus Selector1/4 -> [d_theta301], STG 301/4  "<Rotor angle deviation  d_theta (rad)>"
  301/1 -> Bus Selector1/1, [M301]
  Bus Selector1/1 -> [w301], STG 301/3  "<Rotor speed  wm  (pu)>"
  Bus Selector1/3 -> "Delta w PSS (Kundur) 301 "/1, MB-PSS  301/1  "<Rotor speed deviation  dw (pu)>"
  Real-Imag to Complex/1 -> Complex to Magnitude-Angle/1
  Complex to Magnitude-Angle/1 -> AC4A Excitation System 301/2, [Vt301]
  AC4A Excitation System 301/1 -> 301/2, [EFD301]
  Multiport Switch1/1 -> AC4A Excitation System 301/4, [pss301]
  Bus Selector1/5 -> [theta301]  "<Rotor mechanical angle  theta (deg)>"
  Bus Selector1/2 -> [Pe301]  "<Output active power   Peo (pu)>"
  Bus Selector1/8 -> AC4A Excitation System 301/3  "<Field current  ifd (pu)>"
  STG 301/4 -> [Pm301], 301/1
  Pref/1 -> STG 301/2
  Bus Selector1/9 -> [Q301]  "<Output reactive power  Qeo (pu)>"
  PSS model4/1 -> Sum2/2
  Sum2/1 -> Multiport Switch1/1
  [PSSmodel] -> Sum2/1
  PSS model3/1 -> Multiport Switch1/2
  Sum3/1 -> [Pa301], "Delta Pa PSS 301 "/1  "Pm-Pe"
  "Delta Pa PSS 301 "/1 -> Multiport Switch1/5
  "Delta w PSS (Kundur) 301 "/1 -> Multiport Switch1/4
  [Pm301] -> Sum3/2
  [Pe301] -> Sum3/1
  MB-PSS  301/1 -> Multiport Switch1/3
  STG 301/1 -> Terminator3/1
  STG 301/2 -> Terminator1/1
  STG 301/3 -> Terminator2/1
  connections:
  301/RConn1 -- A/RConn1
  301/RConn2 -- B/RConn1
  301/RConn3 -- C/RConn1

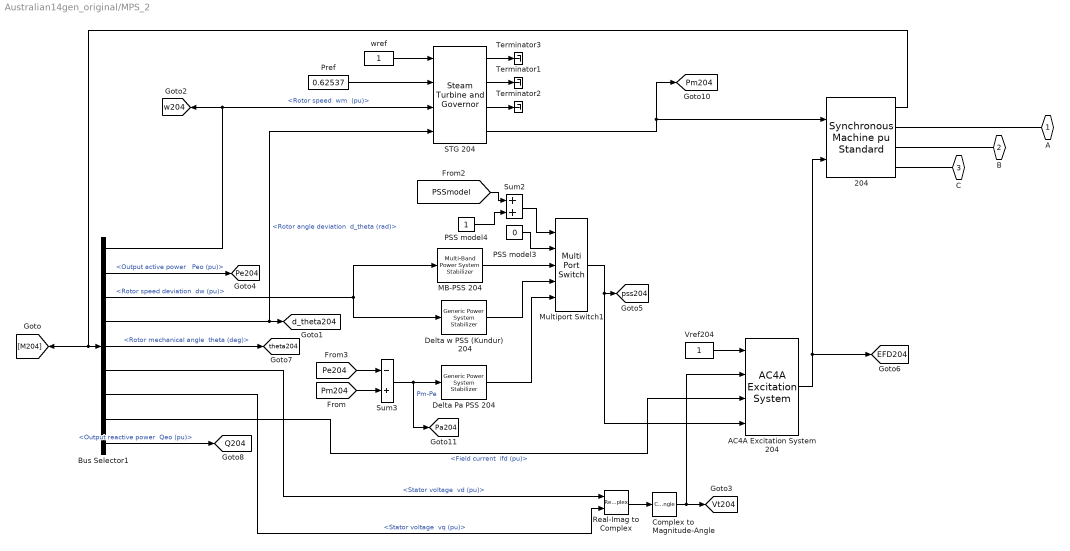
== system Australian14gen_original/MPS_2 ==
  204 : powerlib/Machines/Synchronous Machine pu Standard  PresetModel=No  MechanicalLoad=Mechanical power Pm  ShowDetailedParameters=on  RotorType=Round  Units=per unit standard parameters  MeasurementBus=off  NominalParameters="[G_data(5,2)*1E6  G_data(5,3)*1E3  50]"  Reactances1=[G_data(5,6),G_data(5,8),G_data(5,10),G_data(5,7),G_data(5,12),G_data(5,14),G_data(5,5)]  Reactances2=[G_data(5,6),G_data(5,8),G_data(5,10),G_data(5,7),G_data(5,12),G_data(5,14),G_data(5,5)]  dAxisTimeConstants=Open-circuit  qAxisTimeConstants=Open-circuit  TimeConstants1="[G_data(5,9)  G_data(5,11)  G_data(5,13) G_data(5,15)]"  TimeConstants2="[G_data(5,9)  G_data(5,11)  G_data(5,13) G_data(5,15)]"  TimeConstants3="[  5.9  0.033  0.023  ]"  TimeConstants4=[ 8.0, 0.03, 0.3371, 0.0295 ]  TimeConstants5=[ 1.01, 0.053, 0.1 ]  TimeConstants6=[ 1.3201, 0.023, 1.0, 0.07 ]  TimeConstants7="[  1.01  0.053  0.051266  ]"  TimeConstants8=[ 1.3201, 0.0231, 0.3371, 0.0295 ]  StatorResistance=0  Mechanical="[ G_data(5,4) 0  4 ]"  PolePairs=4  InitialConditions=[0 -39.5945 0.627714 0.627714 0.627714 4.95136 -115.049 124.951 1.44261]  SetSaturation=off  Saturation=[0.6404,0.7127,0.8441,0.9214,0.9956,1.082,1.19,1.316,1.457;0.7,0.7698,0.8872,0.9466,0.9969,1.046,1.1,1.151,1.201]  LoadFlowParameters=[2 1987000000 20000 0 0]  TsPowergui=0  TsBlock=-1  IterativeModel=Forward Euler  IterativeDiscreteModel=Trapezoidal non iterative  BusType=swing  Pref=p(5,3)*1e6  Qref=0  Qmin=-inf  Qmax=inf  PLF=0  QLF=0
      settings: SourceProductName=Simscape Power Systems
  AC4A Excitation System 204 : sps_avr/AC4A Excitation System  Tr=Exc(5,2)  KaTa="[Exc(5,3)   Exc(5,4)]"  VIminmax=[-10 10]  VRminmax=[-4.53 5.64]  TbTc="[Exc(5,5)  Exc(5,6)]"  Kc=0  v0=[1 1.4426]  TsBlock=0
      settings: SourceProductName=Simscape Power Systems  SourceProductBaseCode=PS
  Bus Selector1 : BusSelector  OutputSignals="Mechanical.Rotor speed  wm  (pu),Output active power   Peo (pu),Mechanical.Rotor speed deviation  dw (pu),Mechanical.Rotor angle deviation  d_theta (rad),Mechanical.Rotor mechanical angle  theta (deg),dq0 components.Stator voltage  vd (pu),dq0 components.Stator voltage  vq (pu),dq0 components.Field current  ifd (pu),Output reactive power  Qeo (pu)"
  Complex to Magnitude-Angle : ComplexToMagnitudeAngle  Output=Magnitude
  "Delta Pa PSS 204 " : powerlib/Machines/Generic Power System Stabilizer  Tsensor=15e-3  K=2.5*1.25  Twashout=1  Tleadlag1=[60e-3 1]  Tleadlag2=[0 0]  VSlimits=[-0.15 0.15]  Vinit=0  Plot_On=off  MagdB_On=on  FreqRange=logspace(-2,2,500)
      settings: SourceProductName=Simscape Power Systems  SourceProductBaseCode=PS
  Delta w PSS (Kundur)  204 : powerlib/Machines/Generic Power System Stabilizer  Tsensor=15e-3  K=30  Twashout=10  Tleadlag1=[50e-3 20e-3]  Tleadlag2=[3 5.4]  VSlimits=[-0.15 0.15]  Vinit=0  Plot_On=off  MagdB_On=on  FreqRange=logspace(-2,2,500)
      settings: SourceProductName=Simscape Power Systems  SourceProductBaseCode=PS
  "MB-PSS 204 " : powerlib/Machines/Multi-Band Power System Stabilizer  OperationMode=Simplified settings  Kg=G  GL="[FL  KL]"  GI="[FI  KI]"  GH="[FH  KH]"  GLd=[66 66 9.4]  TcLF=[1.667 2 0 0 0 0 2 2.4 0 0 0 0 1 1]  GId=[66 66 47.6]  TcIF=[1 1 0.25 0.3 0 0 1 1 0.3 0.36 0 0 0 0]  GHd=[66 66 233]  TcHF="[0.01 0.012 0 0 0 0  0.012 0.0144 0 0 0 0 1 1]"  LIM=[.075 .15 .15 .15]  Plot_On=off  MagdB_On=off  FreqRange=logspace(-2,2,500)
      settings: SourceProductName=Simscape Power Systems  SourceProductBaseCode=PS
  Multiport Switch1 : MultiPortSwitch  Inputs=4  InputSameDT=on
  PSS model3 : Constant  Value=0
  PSS model4 : Constant
  Pref : Constant  Value=0.62537
  Real-Imag to Complex : RealImagToComplex
  STG 204 : powerlib/Machines/Steam Turbine and Governor  gentype=Tandem-compound (single mass)  reg1="[ 1  0.05    0 ]"  reg2="[ 0.001  0.15 ]"  reg3="[ -0.1  0.1  0  4.496 ]"  N=3000  turb1="[ 0  10   3.3   0.5   ]"  turb2="[   0   0.36    0.36   0.28   ]"  HA="[ 0.046  1.430  1.465   0.192 ]"  KA="[ 90.44  53.88  64.59   62.94  ]"  DA="[ 0.0115  0.3575  0.3663   0.0137  ]"  ini1=0.62537  ini2=[0.779316,-31.4247]
      settings: SourceProductName=Simscape Power Systems  SourceProductBaseCode=PS
  Sum2 : Sum  SaturateOnIntegerOverflow=on  InputSameDT=on  OutDataTypeStr=Inherit: Same as first input
  Sum3 : Sum  Inputs=-+  SaturateOnIntegerOverflow=on  InputSameDT=on  OutDataTypeStr=Inherit: Same as first input
  Terminator1 : Terminator
  Terminator2 : Terminator
  Terminator3 : Terminator
  Vref204 : Constant
  wref : Constant
  A : PMIOPort  Port=1  Side=Left
  B : PMIOPort  Port=2  Side=Left
  C : PMIOPort  Port=3  Side=Left
  tag scope: EFD204=global, Pa204=global, Pe204=global, Pm204=global, Q204=global, Vt204=global, d_theta204=global, pss204=global, theta204=global, w204=global
  wires:
  Bus Selector1/7 -> Real-Imag to Complex/2  "<Stator voltage  vq (pu)>"
  Bus Selector1/6 -> Real-Imag to Complex/1  "<Stator voltage  vd (pu)>"
  wref/1 -> STG 204/1
  Vref204/1 -> AC4A Excitation System 204/1
  Bus Selector1/4 -> STG 204/4, [d_theta204]  "<Rotor angle deviation  d_theta (rad)>"
  204/1 -> [M204], Bus Selector1/1
  Bus Selector1/1 -> [w204], STG 204/3  "<Rotor speed  wm  (pu)>"
  Bus Selector1/3 -> Delta w PSS (Kundur)  204/1, "MB-PSS 204 "/1  "<Rotor speed deviation  dw (pu)>"
  Real-Imag to Complex/1 -> Complex to Magnitude-Angle/1
  Complex to Magnitude-Angle/1 -> AC4A Excitation System 204/2, [Vt204]
  AC4A Excitation System 204/1 -> [EFD204], 204/2
  Multiport Switch1/1 -> AC4A Excitation System 204/4, [pss204]
  Bus Selector1/5 -> [theta204]  "<Rotor mechanical angle  theta (deg)>"
  Bus Selector1/2 -> [Pe204]  "<Output active power   Peo (pu)>"
  Bus Selector1/8 -> AC4A Excitation System 204/3  "<Field current  ifd (pu)>"
  Bus Selector1/9 -> [Q204]  "<Output reactive power  Qeo (pu)>"
  Pref/1 -> STG 204/2
  STG 204/4 -> [Pm204], 204/1
  PSS model4/1 -> Sum2/2
  Sum2/1 -> Multiport Switch1/1
  [PSSmodel] -> Sum2/1
  PSS model3/1 -> Multiport Switch1/2
  Sum3/1 -> [Pa204], "Delta Pa PSS 204 "/1  "Pm-Pe"
  "Delta Pa PSS 204 "/1 -> Multiport Switch1/5
  Delta w PSS (Kundur)  204/1 -> Multiport Switch1/4
  [Pm204] -> Sum3/2
  [Pe204] -> Sum3/1
  "MB-PSS 204 "/1 -> Multiport Switch1/3
  STG 204/1 -> Terminator3/1
  STG 204/2 -> Terminator1/1
  STG 204/3 -> Terminator2/1
  connections:
  204/RConn1 -- A/RConn1
  204/RConn2 -- B/RConn1
  204/RConn3 -- C/RConn1
